simulink model "V0_2_5_2025_11_18_FullFMS"  (R2025b)
settings: Solver=VariableStepAuto  StartTime=0.0  StopTime=inf  RelTol=1e-3
libraries: opcualib x8
(part 1 of 3)
settings Model: SimulationMode=accelerator  Creator=guilh  LastModifiedBy=guilh

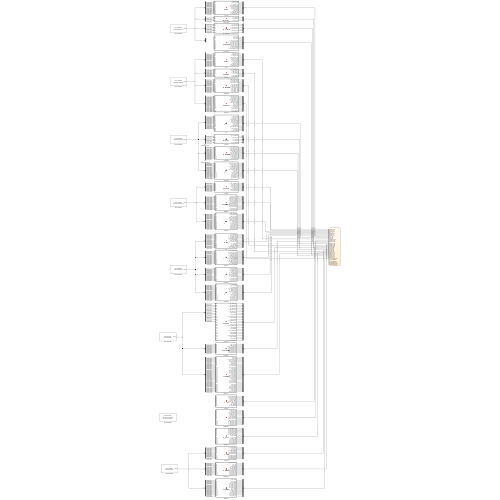
[thumbnail: Simulink's stored preview of the top-level diagram]
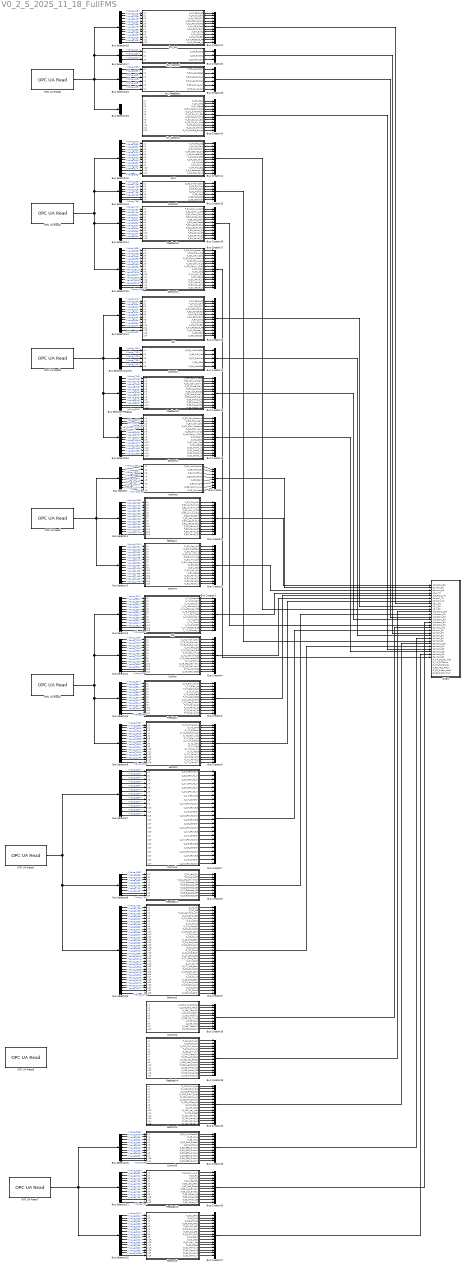
== system V0_2_5_2025_11_18_FullFMS ==
  ASI : MATLAB Function  TreatAsAtomicUnit=on
  Asi : MATLAB Function  TreatAsAtomicUnit=on
  Asi1 : MATLAB Function  TreatAsAtomicUnit=on
  Bus Creator : BusCreator  Inputs=8
  Bus Creator1 : BusCreator  Inputs=13
  Bus Creator10 : BusCreator  Inputs=14
  Bus Creator11 : BusCreator  Inputs=5
  Bus Creator{5,12,14,16,21,24,26} (7 alike) : BusCreator  Inputs=12
  Bus Creator{2,6,13,17,20} (5 alike) : BusCreator  Inputs=15
  Bus Creator15 : BusCreator  Inputs=7
  Bus Creator18 : BusCreator  Inputs=10
  Bus Creator19 : BusCreator  Inputs=14
  Bus Creator22 : BusCreator  Inputs=3
  Bus Creator23 : BusCreator  Inputs=6
  Bus Creator25 : BusCreator  Inputs=11
  Bus Creator27 : BusCreator  Inputs=16
  Bus Creator3 : BusCreator  Inputs=13
  Bus Creator4 : BusCreator  Inputs=13
  Bus Creator7 : BusCreator  Inputs=24
  Bus Creator8 : BusCreator  Inputs=9
  Bus Creator9 : BusCreator  Inputs=33
  Bus Selector : BusSelector  OutputSignals=Value_1062,Value_1072,Value_1082,Value_1094,Value_1104,Value_1114,Value_1124,Value_1134
  Bus Selector/Control : BusSelector  OutputSignals=Value_700,Value_710,Value_720,Value_730,Value_740
  Bus Selector/Feedback : BusSelector  OutputSignals=Value_756,Value_766,Value_776,Value_786,Value_796,Value_806,Value_816,Value_826,Value_836,Value_846,Value_856,Value_866
  Bus Selector1 : BusSelector  OutputSignals=Value_1150,Value_1160,Value_1170,Value_1180,Value_1190,Value_1200,Value_1210,Value_1220,Value_1230,Value_1240,Value_1250,Value_1260,Value_1270
  Bus Selector10 : BusSelector  OutputSignals=Value_885,Value_898,Value_913,Value_926,Value_939,Value_952,Value_965,Value_978,Value_991,Value_1004,Value_1017,Value_1030,Value_1043,Value_1056,Value_1069
  Bus Selector11 : BusSelector  OutputSignals=Value_574,Value_584,Value_594,Value_604,Value_614,Value_624,Value_634,Value_644,Value_654,Value_664,Value_674,Value_684
  Bus Selector12 : BusSelector  OutputSignals=Value_572,Value_582,Value_592,Value_602,Value_612,Value_622,Value_632,Value_642,Value_652,Value_662,Value_672,Value_682
  Bus Selector13 : BusSelector  OutputSignals=Value_698,Value_708,Value_718,Value_728,Value_738,Value_748,Value_758
  Bus Selector14 : BusSelector  OutputSignals=Value_774,Value_784,Value_794,Value_804,Value_814,Value_824,Value_834,Value_844,Value_854,Value_864,Value_874,Value_884
  Bus Selector15 : BusSelector  OutputSignals=Value_905,Value_918,Value_933,Value_946,Value_959,Value_972,Value_985,Value_998,Value_1011,Value_1024,Value_1037,Value_1050,Value_1063,Value_1076,Value_1089
  Bus Selector16 : BusSelector  OutputSignals=Value_215,Value_225,Value_235,Value_245,Value_255,Value_265,Value_275,Value_285,Value_295,Value_305,Value_315,Value_325
  Bus Selector17 : BusSelector  OutputSignals=Value_341,Value_354,Value_367
  Bus Selector18 : BusSelector  OutputSignals=Value_383,Value_393,Value_403,Value_413,Value_423,Value_433
  Bus Selector19 : BusSelector  OutputSignals=signal1,signal2
  Bus Selector2 : BusSelector  OutputSignals=Value_1291,Value_1304,Value_1319,Value_1332,Value_1345,Value_1358,Value_1371,Value_1384,Value_1397,Value_1410,Value_1423,Value_1436,Value_1449,Value_1462,Value_1475
  Bus Selector20 : BusSelector  OutputSignals=Value_566,Value_576,Value_586,Value_596,Value_606,Value_616,Value_626,Value_636,Value_646,Value_656,Value_666
  Bus Selector21 : BusSelector  OutputSignals=Value_682,Value_692,Value_702,Value_712,Value_722,Value_732,Value_742,Value_752,Value_762,Value_772,Value_782,Value_792
  Bus Selector22 : BusSelector  OutputSignals=Value_811,Value_824,Value_839,Value_852,Value_865,Value_878,Value_891,Value_904,Value_917,Value_930,Value_943,Value_956,Value_969,Value_982,Value_995,Value_1008
  Bus Selector3 : BusSelector  OutputSignals=Value_572,Value_582,Value_592,Value_602,Value_612,Value_622,Value_632,Value_642,Value_652,Value_662,Value_672,Value_682,Value_692
  Bus Selector4 : BusSelector  OutputSignals=Value_708,Value_718,Value_728,Value_738,Value_748,Value_758,Value_768,Value_778,Value_788,Value_798,Value_808,Value_818,Value_828
  Bus Selector5 : BusSelector  OutputSignals=Value_844,Value_854,Value_864,Value_874,Value_884,Value_894,Value_904,Value_914,Value_924,Value_934,Value_944,Value_954
  Bus Selector6 : BusSelector  OutputSignals=Value_975,Value_988,Value_1003,Value_1016,Value_1029,Value_1042,Value_1055,Value_1068,Value_1081,Value_1094,Value_1107,Value_1120,Value_1133,Value_1146,Value_1159
  Bus Selector7 : BusSelector  OutputSignals=Value_527,Value_537,Value_547,Value_557,Value_567,Value_577,Value_587,Value_597,Value_607,Value_617,Value_627,Value_637
  Bus Selector8 : BusSelector  OutputSignals=Value_653,Value_663,Value_673,Value_683,Value_693,Value_703,Value_713,Value_723,Value_733
  Bus Selector9 : BusSelector  OutputSignals=Value_752,Value_765,Value_780,Value_793,Value_806,Value_819,Value_832,Value_845,Value_858,Value_871,Value_884,Value_897,Value_910,Value_923,Value_936,Value_949,Value_962,Value_975,Value_988,Value_1001,Value_1014,Value_1027,Value_1040,Value_1053,Value_1066,Value_1079,Value_1092,Value_1105,Value_1118,Value_1131,Value_1144,Value_1157,Value_1170
  Chart : Stateflow chart  TreatAsAtomicUnit=on
      settings: PortSchema="{\"entries\":[{\"content\":{\"sides\":[{\"content\":{\"connectorIds\":[\"In2\",\"In1\",\"In3\",\"In4\",\"In6\",\"In5\",\"In7\",\"In8\",\"In9\",\"In10\",\"In11\",\"In12\",\"In13\",\"In14\",\"In15\",\"In16\",\"In17\",\"In18\",\"In19\",\"In20\",\"In21\",\"In22\",\"In23\",\"In24\",\"In25\",\"In26\",\"In27\",\"In28\",\"In29\",\"In30\",\"In31\",\"In32\",\"In33\",\"In34\"]},\"type\":\"ConnectorPlacement.EquallySpacedRectSide\",\"uuid\":\"e54bf7d4-7c7d-41d9-a8b8-f479ac319a99\"},{\"content\":{\"side\":\"RIGHT\"},\"type\":\"ConnectorPlacement.EquallySpacedRectSide\",\"uuid\":\"d3c20706-71bd-4e26-b40f-0ee7e71b06ee\"},{\"content\":{\"side\":\"TOP\"},\"type\":\"ConnectorPlacement.EquallySpacedRectSide\",\"uuid\":\"ecfb6920-e95b-4ed8-99f9-df5ce878328e\"}]},\"type\":\"ConnectorPlacement.EquallySpacedConnector\",\"uuid\":\"2e714192-4eea-4e1a-8945-7c827feed48f\"}],\"packageUris\":[\"http://schema.mathworks.com/mf0/Connector/R2020b\"],\"version\":\"1.0\"}"
  Control : MATLAB Function  TreatAsAtomicUnit=on
  Control1 : MATLAB Function  TreatAsAtomicUnit=on
  Control2 : MATLAB Function  TreatAsAtomicUnit=on
  Control3 : MATLAB Function  TreatAsAtomicUnit=on
  Control4 : MATLAB Function  TreatAsAtomicUnit=on
  Control5 : MATLAB Function  TreatAsAtomicUnit=on
  Feedback : MATLAB Function  TreatAsAtomicUnit=on
  Feedback1 : MATLAB Function  TreatAsAtomicUnit=on
  Feedback2 : MATLAB Function  TreatAsAtomicUnit=on
  Feedback3 : MATLAB Function  TreatAsAtomicUnit=on
  Feedback4 : MATLAB Function  TreatAsAtomicUnit=on
  Feedback5 : MATLAB Function  TreatAsAtomicUnit=on
  OPC UA Read : opcualib/OPC UA Read  SelectedServer=AAS OPC Distribution  ServerList=AAS OPC Distribution  NodeList={ '1', 'Value', '6', '1062', '1'; '2', 'Value', '6', '1072', '1'; '3', 'Value', '6', '1082', '1'; '4', 'Value', '6', '1094', '1'; '5', 'Value', '6', '1104', '1'; '6', 'Value', '6', '1114', '1'; '7', 'Value', '6', '1124', '1'; '8', 'Value', '6', '1134', '1'; '9', 'Value', '6', '1150', '1'; '10', 'Value', '6', '1160', '1'; '11', 'Value', '6', '1170', '1'; '12', 'Value', '6', '1180', '1'; '13', 'Value', '6', '1190', '1'; '14', 'Value', '6', '1200', '1'; '15', 'Value', '6', '1210', '1'; '16', 'Value', '6', '1220', '1'; '17', 'Value', '6', '1230', '1'; '18', 'Value', '6', '1240', '1'; '19', 'Value', '6', '1250', '1'; '20', 'Value', '6', '1260', '1'; '21', 'Value', '6', '1270', '1'; '22', 'Value', '6', '1291', '1'; '23', 'Value', '6', '1304', '1'; '24', 'Value', '6', '1319', '1'; '25', 'Value', '6', '1332', '1'; '26', 'Value', '6', '1345', '1'; '27', 'Value', '6', '1358', '1'; '28', 'Value', '6', '1371', '1'; '29', 'Value', '6', '1384', '1'; '30', 'Value', '6', '1397', '1'; '31', 'Value', '6', '1410', '1'; '32', 'Value', '6', '1423', '1'; '33', 'Value', '6', '1436', '1'; '34', 'Value', '6', '1449', '1'; '35', 'Value', '6', '1462', '1'; '36', 'Value', '6', '1475', '1' }  ShowQualityPort=off  ShowTimestampPort=off  ShowTimestampPortAs=Seconds since start  SampleTime=-1
  OPC UA Read1 : opcualib/OPC UA Read  SelectedServer=AAS OPC Testing  ServerList=AAS OPC Testing  NodeList={ '1', 'Value', '6', '572', '1'; '2', 'Value', '6', '582', '1'; '3', 'Value', '6', '592', '1'; '4', 'Value', '6', '602', '1'; '5', 'Value', '6', '612', '1'; '6', 'Value', '6', '622', '1'; '7', 'Value', '6', '632', '1'; '8', 'Value', '6', '642', '1'; '9', 'Value', '6', '652', '1'; '10', 'Value', '6', '662', '1'; '11', 'Value', '6', '672', '1'; '12', 'Value', '6', '682', '1'; '13', 'Value', '6', '692', '1'; '14', 'Value', '6', '708', '1'; '15', 'Value', '6', '718', '1'; '16', 'Value', '6', '728', '1'; '17', 'Value', '6', '738', '1'; '18', 'Value', '6', '748', '1'; '19', 'Value', '6', '758', '1'; '20', 'Value', '6', '768', '1'; '21', 'Value', '6', '778', '1'; '22', 'Value', '6', '788', '1'; '23', 'Value', '6', '798', '1'; '24', 'Value', '6', '808', '1'; '25', 'Value', '6', '818', '1'; '26', 'Value', '6', '828', '1'; '27', 'Value', '6', '844', '1'; '28', 'Value', '6', '854', '1'; '29', 'Value', '6', '864', '1'; '30', 'Value', '6', '874', '1'; '31', 'Value', '6', '884', '1'; '32', 'Value', '6', '894', '1'; '33', 'Value', '6', '904', '1'; '34', 'Value', '6', '914', '1'; '35', 'Value', '6', '924', '1'; '36', 'Value', '6', '934', '1'; '37', 'Value', '6', '944', '1'; '38', 'Value', '6', '954', '1'; '39', 'Value', '6', '975', '1'; '40', 'Value', '6', '988', '1'; '41', 'Value', '6', '1003', '1'; '42', 'Value', '6', '1016', '1'; '43', 'Value', '6', '1029', '1'; '44', 'Value', '6', '1042', '1'; '45', 'Value', '6', '1055', '1'; '46', 'Value', '6', '1068', '1'; '47', 'Value', '6', '1081', '1'; '48', 'Value', '6', '1094', '1'; '49', 'Value', '6', '1107', '1'; '50', 'Value', '6', '1120', '1'; '51', 'Value', '6', '1133', '1'; '52', 'Value', '6', '1146', '1'; '53', 'Value', '6', '1159', '1' }  ShowQualityPort=off  ShowTimestampPort=off  ShowTimestampPortAs=Seconds since start  SampleTime=-1
  OPC UA Read2 : opcualib/OPC UA Read  SelectedServer=AAS OPC Master  ServerList=AAS OPC Master  NodeList={ '1', 'Value', '6', '527', '1'; '2', 'Value', '6', '537', '1'; '3', 'Value', '6', '547', '1'; '4', 'Value', '6', '557', '1'; '5', 'Value', '6', '567', '1'; '6', 'Value', '6', '577', '1'; '7', 'Value', '6', '587', '1'; '8', 'Value', '6', '597', '1'; '9', 'Value', '6', '607', '1'; '10', 'Value', '6', '617', '1'; '11', 'Value', '6', '627', '1'; '12', 'Value', '6', '637', '1'; '13', 'Value', '6', '653', '1'; '14', 'Value', '6', '663', '1'; '15', 'Value', '6', '673', '1'; '16', 'Value', '6', '683', '1'; '17', 'Value', '6', '693', '1'; '18', 'Value', '6', '703', '1'; '19', 'Value', '6', '713', '1'; '20', 'Value', '6', '723', '1'; '21', 'Value', '6', '733', '1'; '22', 'Value', '6', '752', '1'; '23', 'Value', '6', '765', '1'; '24', 'Value', '6', '780', '1'; '25', 'Value', '6', '793', '1'; '26', 'Value', '6', '806', '1'; '27', 'Value', '6', '819', '1'; '28', 'Value', '6', '832', '1'; '29', 'Value', '6', '845', '1'; '30', 'Value', '6', '858', '1'; '31', 'Value', '6', '871', '1'; '32', 'Value', '6', '884', '1'; '33', 'Value', '6', '897', '1'; '34', 'Value', '6', '910', '1'; '35', 'Value', '6', '923', '1'; '36', 'Value', '6', '936', '1'; '37', 'Value', '6', '949', '1'; '38', 'Value', '6', '962', '1'; '39', 'Value', '6', '975', '1'; '40', 'Value', '6', '988', '1'; '41', 'Value', '6', '1001', '1'; '42', 'Value', '6', '1014', '1'; '43', 'Value', '6', '1027', '1'; '44', 'Value', '6', '1040', '1'; '45', 'Value', '6', '1053', '1'; '46', 'Value', '6', '1066', '1'; '47', 'Value', '6', '1079', '1'; '48', 'Value', '6', '1092', '1'; '49', 'Value', '6', '1105', '1'; '50', 'Value', '6', '1118', '1'; '51', 'Value', '6', '1131', '1'; '52', 'Value', '6', '1144', '1'; '53', 'Value', '6', '1157', '1'; '54', 'Value', '6', '1170', '1' }  ShowQualityPort=off  ShowTimestampPort=off  ShowTimestampPortAs=Seconds since start  SampleTime=-1
  OPC UA Read3 : opcualib/OPC UA Read  SelectedServer=AAS OPC Handling1  ServerList=AAS OPC Handling1  NodeList={ '1', 'Value', '6', '574', '1'; '2', 'Value', '6', '584', '1'; '3', 'Value', '6', '594', '1'; '4', 'Value', '6', '604', '1'; '5', 'Value', '6', '614', '1'; '6', 'Value', '6', '624', '1'; '7', 'Value', '6', '634', '1'; '8', 'Value', '6', '644', '1'; '9', 'Value', '6', '654', '1'; '10', 'Value', '6', '664', '1'; '11', 'Value', '6', '674', '1'; '12', 'Value', '6', '684', '1'; '13', 'Value', '6', '700', '1'; '14', 'Value', '6', '710', '1'; '15', 'Value', '6', '720', '1'; '16', 'Value', '6', '730', '1'; '17', 'Value', '6', '740', '1'; '18', 'Value', '6', '756', '1'; '19', 'Value', '6', '766', '1'; '20', 'Value', '6', '776', '1'; '21', 'Value', '6', '786', '1'; '22', 'Value', '6', '796', '1'; '23', 'Value', '6', '806', '1'; '24', 'Value', '6', '816', '1'; '25', 'Value', '6', '826', '1'; '26', 'Value', '6', '836', '1'; '27', 'Value', '6', '846', '1'; '28', 'Value', '6', '856', '1'; '29', 'Value', '6', '866', '1'; '30', 'Value', '6', '885', '1'; '31', 'Value', '6', '898', '1'; '32', 'Value', '6', '913', '1'; '33', 'Value', '6', '926', '1'; '34', 'Value', '6', '939', '1'; '35', 'Value', '6', '952', '1'; '36', 'Value', '6', '965', '1'; '37', 'Value', '6', '978', '1'; '38', 'Value', '6', '991', '1'; '39', 'Value', '6', '1004', '1'; '40', 'Value', '6', '1017', '1'; '41', 'Value', '6', '1030', '1'; '42', 'Value', '6', '1043', '1'; '43', 'Value', '6', '1056', '1'; '44', 'Value', '6', '1069', '1' }  ShowQualityPort=off  ShowTimestampPort=off  ShowTimestampPortAs=Seconds since start  SampleTime=-1
  OPC UA Read4 : opcualib/OPC UA Read  SelectedServer=AAS OPC Handling2  ServerList=AAS OPC Handling2  NodeList={ '1', 'Value', '6', '572', '1'; '2', 'Value', '6', '582', '1'; '3', 'Value', '6', '592', '1'; '4', 'Value', '6', '602', '1'; '5', 'Value', '6', '612', '1'; '6', 'Value', '6', '622', '1'; '7', 'Value', '6', '632', '1'; '8', 'Value', '6', '642', '1'; '9', 'Value', '6', '652', '1'; '10', 'Value', '6', '662', '1'; '11', 'Value', '6', '672', '1'; '12', 'Value', '6', '682', '1'; '13', 'Value', '6', '698', '1'; '14', 'Value', '6', '708', '1'; '15', 'Value', '6', '718', '1'; '16', 'Value', '6', '728', '1'; '17', 'Value', '6', '738', '1'; '18', 'Value', '6', '748', '1'; '19', 'Value', '6', '758', '1'; '20', 'Value', '6', '774', '1'; '21', 'Value', '6', '784', '1'; '22', 'Value', '6', '794', '1'; '23', 'Value', '6', '804', '1'; '24', 'Value', '6', '814', '1'; '25', 'Value', '6', '824', '1'; '26', 'Value', '6', '834', '1'; '27', 'Value', '6', '844', '1'; '28', 'Value', '6', '854', '1'; '29', 'Value', '6', '864', '1'; '30', 'Value', '6', '874', '1'; '31', 'Value', '6', '884', '1'; '32', 'Value', '6', '905', '1'; '33', 'Value', '6', '918', '1'; '34', 'Value', '6', '933', '1'; '35', 'Value', '6', '946', '1'; '36', 'Value', '6', '959', '1'; '37', 'Value', '6', '972', '1'; '38', 'Value', '6', '985', '1'; '39', 'Value', '6', '998', '1'; '40', 'Value', '6', '1011', '1'; '41', 'Value', '6', '1024', '1'; '42', 'Value', '6', '1037', '1'; '43', 'Value', '6', '1050', '1'; '44', 'Value', '6', '1063', '1'; '45', 'Value', '6', '1076', '1'; '46', 'Value', '6', '1089', '1' }  ShowQualityPort=off  ShowTimestampPort=off  ShowTimestampPortAs=Seconds since start  SampleTime=-1
  OPC UA Read5 : opcualib/OPC UA Read  SelectedServer=AAS OPC Processing  ServerList=AAS OPC Processing  NodeList={}  ShowQualityPort=on  ShowTimestampPort=on  ShowTimestampPortAs=Seconds since start  SampleTime=-1
  OPC UA Read6 : opcualib/OPC UA Read  SelectedServer=Node-RED OPCUA  ServerList=Node-RED OPCUA  NodeList={ '1', 'Value', '6', '215', '1'; '2', 'Value', '6', '225', '1'; '3', 'Value', '6', '235', '1'; '4', 'Value', '6', '245', '1'; '5', 'Value', '6', '255', '1'; '6', 'Value', '6', '265', '1'; '7', 'Value', '6', '275', '1'; '8', 'Value', '6', '285', '1'; '9', 'Value', '6', '295', '1'; '10', 'Value', '6', '305', '1'; '11', 'Value', '6', '315', '1'; '12', 'Value', '6', '325', '1'; '13', 'Value', '6', '341', '1'; '14', 'Value', '6', '354', '1'; '15', 'Value', '6', '367', '1'; '16', 'Value', '6', '383', '1'; '17', 'Value', '6', '393', '1'; '18', 'Value', '6', '403', '1'; '19', 'Value', '6', '413', '1'; '20', 'Value', '6', '423', '1'; '21', 'Value', '6', '433', '1' }  ShowQualityPort=off  ShowTimestampPort=off  ShowTimestampPortAs=Seconds since start  SampleTime=-1
  OPC UA Read7 : opcualib/OPC UA Read  SelectedServer=AAS OPC Sorting  ServerList=AAS OPC Sorting  NodeList={ '1', 'Value', '6', '566', '1'; '2', 'Value', '6', '576', '1'; '3', 'Value', '6', '586', '1'; '4', 'Value', '6', '596', '1'; '5', 'Value', '6', '606', '1'; '6', 'Value', '6', '616', '1'; '7', 'Value', '6', '626', '1'; '8', 'Value', '6', '636', '1'; '9', 'Value', '6', '646', '1'; '10', 'Value', '6', '656', '1'; '11', 'Value', '6', '666', '1'; '12', 'Value', '6', '682', '1'; '13', 'Value', '6', '692', '1'; '14', 'Value', '6', '702', '1'; '15', 'Value', '6', '712', '1'; '16', 'Value', '6', '722', '1'; '17', 'Value', '6', '732', '1'; '18', 'Value', '6', '742', '1'; '19', 'Value', '6', '752', '1'; '20', 'Value', '6', '762', '1'; '21', 'Value', '6', '772', '1'; '22', 'Value', '6', '782', '1'; '23', 'Value', '6', '792', '1'; '24', 'Value', '6', '811', '1'; '25', 'Value', '6', '824', '1'; '26', 'Value', '6', '839', '1'; '27', 'Value', '6', '852', '1'; '28', 'Value', '6', '865', '1'; '29', 'Value', '6', '878', '1'; '30', 'Value', '6', '891', '1'; '31', 'Value', '6', '904', '1'; '32', 'Value', '6', '917', '1'; '33', 'Value', '6', '930', '1'; '34', 'Value', '6', '943', '1'; '35', 'Value', '6', '956', '1'; '36', 'Value', '6', '969', '1'; '37', 'Value', '6', '982', '1'; '38', 'Value', '6', '995', '1'; '39', 'Value', '6', '1008', '1' }  ShowQualityPort=off  ShowTimestampPort=off  ShowTimestampPortAs=Seconds since start  SampleTime=-1
  Sensors : MATLAB Function  TreatAsAtomicUnit=on
  Sensors1 : MATLAB Function  TreatAsAtomicUnit=on
  Sensors2 : MATLAB Function  TreatAsAtomicUnit=on
  Sensors3 : MATLAB Function  TreatAsAtomicUnit=on
  Sensors4 : MATLAB Function  TreatAsAtomicUnit=on
  Sensors5 : MATLAB Function  TreatAsAtomicUnit=on
  controls : MATLAB Function  TreatAsAtomicUnit=on
  fcn_Asi : MATLAB Function  TreatAsAtomicUnit=on
  fcn_Control : MATLAB Function  TreatAsAtomicUnit=on
  fcn_Feedback : MATLAB Function  TreatAsAtomicUnit=on
  fcn_Sensors : MATLAB Function  TreatAsAtomicUnit=on
  feedback : MATLAB Function  TreatAsAtomicUnit=on
  sensors : MATLAB Function  TreatAsAtomicUnit=on
  wires:
  OPC UA Read/1 -> Bus Selector2/1, Bus Selector/1, Bus Selector1/1
  Bus Selector/1 -> controls/1(u1)  "<Value_1062>"
  Bus Selector/2 -> controls/2(u2)  "<Value_1072>"
  Bus Selector/3 -> controls/3(u3)  "<Value_1082>"
  Bus Selector/4 -> controls/4(u4)  "<Value_1094>"
  Bus Selector/5 -> controls/5(u5)  "<Value_1104>"
  Bus Selector/6 -> controls/6(u6)  "<Value_1114>"
  Bus Selector/7 -> controls/7(u7)  "<Value_1124>"
  Bus Selector/8 -> controls/8(u8)  "<Value_1134>"
  Bus Selector1/11 -> feedback/11(u11)  "<Value_1250>"
  Bus Selector1/12 -> feedback/12(u12)  "<Value_1260>"
  Bus Selector1/13 -> feedback/13(u13)  "<Value_1270>"
  Bus Selector1/1 -> feedback/1(u1)  "<Value_1150>"
  Bus Selector1/2 -> feedback/2(u2)  "<Value_1160>"
  Bus Selector1/3 -> feedback/3(u3)  "<Value_1170>"
  Bus Selector1/4 -> feedback/4(u4)  "<Value_1180>"
  Bus Selector1/5 -> feedback/5(u5)  "<Value_1190>"
  Bus Selector1/6 -> feedback/6(u6)  "<Value_1200>"
  Bus Selector1/7 -> feedback/7(u7)  "<Value_1210>"
  Bus Selector1/8 -> feedback/8(u8)  "<Value_1220>"
  Bus Selector1/9 -> feedback/9(u9)  "<Value_1230>"
  Bus Selector1/10 -> feedback/10(u10)  "<Value_1240>"
  Bus Selector2/1 -> sensors/1(u1)  "<Value_1291>"
  Bus Selector2/2 -> sensors/2(u2)  "<Value_1304>"
  Bus Selector2/3 -> sensors/3(u3)  "<Value_1319>"
  Bus Selector2/4 -> sensors/4(u4)  "<Value_1332>"
  Bus Selector2/5 -> sensors/5(u5)  "<Value_1345>"
  Bus Selector2/6 -> sensors/6(u6)  "<Value_1358>"
  Bus Selector2/7 -> sensors/7(u7)  "<Value_1371>"
  Bus Selector2/8 -> sensors/8(u8)  "<Value_1384>"
  Bus Selector2/9 -> sensors/9(u9)  "<Value_1397>"
  Bus Selector2/10 -> sensors/10(u10)  "<Value_1410>"
  Bus Selector2/11 -> sensors/11(u11)  "<Value_1423>"
  Bus Selector2/12 -> sensors/12(u12)  "<Value_1436>"
  Bus Selector2/13 -> sensors/13(u13)  "<Value_1449>"
  Bus Selector2/14 -> sensors/14(u14)  "<Value_1462>"
  Bus Selector2/15 -> sensors/15(u15)  "<Value_1475>"
  OPC UA Read1/1 -> Bus Selector6/1, Bus Selector5/1, Bus Selector3/1, Bus Selector4/1
  Bus Selector3/1 -> ASI/1(u1)  "<Value_572>"
  Bus Selector3/2 -> ASI/2(u2)  "<Value_582>"
  Bus Selector3/3 -> ASI/3(u3)  "<Value_592>"
  Bus Selector3/4 -> ASI/4(u4)  "<Value_602>"
  Bus Selector3/5 -> ASI/5(u5)  "<Value_612>"
  Bus Selector3/6 -> ASI/6(u6)  "<Value_622>"
  Bus Selector3/7 -> ASI/7(u7)  "<Value_632>"
  Bus Selector3/8 -> ASI/8(u8)  "<Value_642>"
  Bus Selector3/9 -> ASI/9(u9)  "<Value_652>"
  Bus Selector3/10 -> ASI/10(u10)  "<Value_662>"
  Bus Selector3/11 -> ASI/11(u11)  "<Value_672>"
  Bus Selector3/12 -> ASI/12(u12)  "<Value_682>"
  Bus Selector3/13 -> ASI/13(u13)  "<Value_692>"
  Bus Selector4/1 -> Control/1(u1)  "<Value_708>"
  Bus Selector4/2 -> Control/2(u2)  "<Value_718>"
  Bus Selector4/3 -> Control/3(u3)  "<Value_728>"
  Bus Selector4/4 -> Control/4(u4)  "<Value_738>"
  Bus Selector4/5 -> Control/5(u5)  "<Value_748>"
  Bus Selector4/6 -> Control/6(u6)  "<Value_758>"
  Bus Selector4/7 -> Control/7(u7)  "<Value_768>"
  Bus Selector4/8 -> Control/8(u8)  "<Value_778>"
  Bus Selector4/9 -> Control/9(u9)  "<Value_788>"
  Bus Selector4/10 -> Control/10(u10)  "<Value_798>"
  Bus Selector4/11 -> Control/11(u11)  "<Value_808>"
  Bus Selector4/12 -> Control/12(u12)  "<Value_818>"
  Bus Selector4/13 -> Control/13(u13)  "<Value_828>"
  Bus Selector5/1 -> Feedback/1(u1)  "<Value_844>"
  Bus Selector5/2 -> Feedback/2(u2)  "<Value_854>"
  Bus Selector5/3 -> Feedback/3(u3)  "<Value_864>"
  Bus Selector5/4 -> Feedback/4(u4)  "<Value_874>"
  Bus Selector5/5 -> Feedback/5(u5)  "<Value_884>"
  Bus Selector5/6 -> Feedback/6(u6)  "<Value_894>"
  Bus Selector5/7 -> Feedback/7(u7)  "<Value_904>"
  Bus Selector5/8 -> Feedback/8(u8)  "<Value_914>"
  Bus Selector5/9 -> Feedback/9(u9)  "<Value_924>"
  Bus Selector5/10 -> Feedback/10(u10)  "<Value_934>"
  Bus Selector5/11 -> Feedback/11(u11)  "<Value_944>"
  Bus Selector5/12 -> Feedback/12(u12)  "<Value_954>"
  Bus Selector6/1 -> Sensors/1(u1)  "<Value_975>"
  Bus Selector6/2 -> Sensors/2(u2)  "<Value_988>"
  Bus Selector6/3 -> Sensors/3(u3)  "<Value_1003>"
  Bus Selector6/4 -> Sensors/4(u4)  "<Value_1016>"
  Bus Selector6/5 -> Sensors/5(u5)  "<Value_1029>"
  Bus Selector6/6 -> Sensors/6(u6)  "<Value_1042>"
  Bus Selector6/7 -> Sensors/7(u7)  "<Value_1055>"
  Bus Selector6/8 -> Sensors/8(u8)  "<Value_1068>"
  Bus Selector6/9 -> Sensors/9(u9)  "<Value_1081>"
  Bus Selector6/10 -> Sensors/10(u10)  "<Value_1094>"
  Bus Selector6/11 -> Sensors/11(u11)  "<Value_1107>"
  Bus Selector6/12 -> Sensors/12(u12)  "<Value_1120>"
  Bus Selector6/13 -> Sensors/13(u13)  "<Value_1133>"
  Bus Selector6/14 -> Sensors/14(u14)  "<Value_1146>"
  Bus Selector6/15 -> Sensors/15(u15)  "<Value_1159>"
  controls/1(C_85_Initialization) -> Bus Creator/1
  controls/2(C_85_Part_Del) -> Bus Creator/2
  controls/3(C_82_Profibus) -> Bus Creator/3
  controls/4(C_83_RQ_Parts) -> Bus Creator/4
  controls/5(C_85_Start) -> Bus Creator/5
  controls/6(C_85_Single) -> Bus Creator/6
  controls/7(C_85_Continuous) -> Bus Creator/7
  controls/8(C_85_Counted) -> Bus Creator/8
  feedback/1(F_82_Pist_Adv) -> Bus Creator1/1
  feedback/2(F_82_Suction_On) -> Bus Creator1/2
  feedback/3(F_82_Suction_Off) -> Bus Creator1/3
  feedback/4(F_82_Arm_2_Del) -> Bus Creator1/4
  feedback/5(F_82_Arm_2_Mag) -> Bus Creator1/5
  feedback/6(F_83_Led_Start) -> Bus Creator1/6
  feedback/7(F_83_Led_Reset) -> Bus Creator1/7
  feedback/8(F_83_Led_Extra1) -> Bus Creator1/8
  feedback/9(F_83_Led_Extra2) -> Bus Creator1/9
  feedback/10(F_83_Panel_O4) -> Bus Creator1/10
  feedback/11(F_83_Panel_O5) -> Bus Creator1/11
  feedback/12(F_83_Panel_O6) -> Bus Creator1/12
  feedback/13(F_83_Panel_O7) -> Bus Creator1/13
  sensors/1(O_80_Mag_Full) -> Bus Creator2/1
  sensors/2(O_80_Pist_Back) -> Bus Creator2/2
  sensors/3(O_80_Pist_Fwd) -> Bus Creator2/3
  sensors/4(O_80_Part_Stuck) -> Bus Creator2/4
  sensors/5(O_80_Arm_Mag) -> Bus Creator2/5
  sensors/6(O_80_Arm_Del) -> Bus Creator2/6
  sensors/7(O_80_Mag_Empty) -> Bus Creator2/7
  sensors/8(O_81_Start) -> Bus Creator2/8
  sensors/9(O_81_Stop) -> Bus Creator2/9
  sensors/10(O_81_Key_Pos) -> Bus Creator2/10
  sensors/11(O_81_Reset) -> Bus Creator2/11
  sensors/12(O_81_Panel_I4) -> Bus Creator2/12
  sensors/13(O_81_Panel_I5) -> Bus Creator2/13
  sensors/14(O_81_Panel_I6) -> Bus Creator2/14
  sensors/15(O_81_Panel_I7) -> Bus Creator2/15
  ASI/1(A_74_Request) -> Bus Creator3/1
  ASI/2(A_74_No_Cart) -> Bus Creator3/2
  ASI/3(A_74_Cart_Full) -> Bus Creator3/3
  ASI/4(A_74_CRoute_Out) -> Bus Creator3/4
  ASI/5(A_74_CRoute_In80) -> Bus Creator3/5
  ASI/6(A_73_TestCartID) -> Bus Creator3/6
  ASI/7(A_74_Cart_Stat) -> Bus Creator3/7
  ASI/8(A_74_Cart_Next) -> Bus Creator3/8
  ASI/9(A_74_Optic) -> Bus Creator3/9
  ASI/10(A_74_Count) -> Bus Creator3/10
  ASI/11(A_74_Pist_Bck) -> Bus Creator3/11
  ASI/12(A_74_Release_FB) -> Bus Creator3/12
  ASI/13(A_74_CRoute_In) -> Bus Creator3/13
  Control/1(C_75_Initialization) -> Bus Creator4/1
  Control/2(C_75_ID_Delivery1) -> Bus Creator4/2
  Control/3(C_75_ID_Delivery2) -> Bus Creator4/3
  Control/4(C_75_Part_Del) -> Bus Creator4/4
  Control/5(C_75_RQ_Part_Del) -> Bus Creator4/5
  Control/6(C_75_RQ_Wrong) -> Bus Creator4/6
  Control/7(C_75_Identified80) -> Bus Creator4/7
  Control/8(C_75_Requested80) -> Bus Creator4/8
  Control/9(C_72_Profibus) -> Bus Creator4/9
  Control/10(C_75_RQ_Delivery1) -> Bus Creator4/10
  Control/11(C_75_RQ_Delivery2) -> Bus Creator4/11
  Control/12(C_75_Identified) -> Bus Creator4/12
  Control/13(C_75_Requested) -> Bus Creator4/13
  Feedback/1(F_72_Elev_Down) -> Bus Creator5/1
  Feedback/2(F_72_Elev_Up) -> Bus Creator5/2
  Feedback/3(F_72_Eject_Part) -> Bus Creator5/3
  Feedback/4(F_72_Air_On) -> Bus Creator5/4
  Feedback/5(F_73_Led_Start) -> Bus Creator5/5
  Feedback/6(F_73_Led_Reset) -> Bus Creator5/6
  Feedback/7(F_73_Led_Extra1) -> Bus Creator5/7
  Feedback/8(F_73_Led_Extra2) -> Bus Creator5/8
  Feedback/9(F_73_Panel_O4) -> Bus Creator5/9
  Feedback/10(F_73_Panel_O5) -> Bus Creator5/10
  Feedback/11(F_73_Panel_O6) -> Bus Creator5/11
  Feedback/12(F_73_Panel_O7) -> Bus Creator5/12
  Sensors/1(O_70_SInductive) -> Bus Creator6/1
  Sensors/2(O_70_SPart) -> Bus Creator6/2
  Sensors/3(O_70_SStation) -> Bus Creator6/3
  Sensors/4(O_70_SPart_Height) -> Bus Creator6/4
  Sensors/5(O_70_Elev_High) -> Bus Creator6/5
  Sensors/6(O_70_Elev_Low) -> Bus Creator6/6
  Sensors/7(O_70_Pist_Back) -> Bus Creator6/7
  Sensors/8(O_71_Start) -> Bus Creator6/8
  Sensors/9(O_71_Stop) -> Bus Creator6/9
  Sensors/10(O_71_Key_Pos) -> Bus Creator6/10
  Sensors/11(O_71_Reset) -> Bus Creator6/11
  Sensors/12(O_71_Panel_I4) -> Bus Creator6/12
  Sensors/13(O_71_Panel_I5) -> Bus Creator6/13
  Sensors/14(O_71_Panel_I6) -> Bus Creator6/14
  Sensors/15(O_71_Panel_I7) -> Bus Creator6/15
  Bus Creator/1 -> Chart/1(Control_80)
  Bus Creator1/1 -> Chart/2(Actuators_80)
  Bus Creator2/1 -> Chart/3(Sensors_80)
  Bus Creator6/1 -> Chart/7(Sensors_70)
  Bus Creator5/1 -> Chart/6(Actuators_70)
  Bus Creator4/1 -> Chart/5(Control_70)
  Bus Creator3/1 -> Chart/4(AS_i_70)
  OPC UA Read2/1 -> Bus Selector9/1, Bus Selector8/1, Bus Selector7/1
  Bus Selector7/1 -> Control1/1(u1)  "<Value_527>"
  Bus Selector7/2 -> Control1/2(u2)  "<Value_537>"
  Bus Selector7/3 -> Control1/3(u3)  "<Value_547>"
  Bus Selector7/4 -> Control1/4(u4)  "<Value_557>"
  Bus Selector7/5 -> Control1/5(u5)  "<Value_567>"
  Bus Selector7/6 -> Control1/6(u6)  "<Value_577>"
  Bus Selector7/7 -> Control1/7(u7)  "<Value_587>"
  Bus Selector7/8 -> Control1/8(u8)  "<Value_597>"
  Bus Selector7/9 -> Control1/9(u9)  "<Value_607>"
  Bus Selector7/10 -> Control1/10(u10)  "<Value_617>"
  Bus Selector7/11 -> Control1/11(u11)  "<Value_627>"
  Bus Selector7/12 -> Control1/12(u12)  "<Value_637>"
  Bus Selector8/1 -> Feedback1/1(u1)  "<Value_653>"
  Bus Selector8/2 -> Feedback1/2(u2)  "<Value_663>"
  Bus Selector8/3 -> Feedback1/3(u3)  "<Value_673>"
  Bus Selector8/4 -> Feedback1/4(u4)  "<Value_683>"
  Bus Selector8/5 -> Feedback1/5(u5)  "<Value_693>"
  Bus Selector8/6 -> Feedback1/6(u6)  "<Value_703>"
  Bus Selector8/7 -> Feedback1/7(u7)  "<Value_713>"
  Bus Selector8/8 -> Feedback1/8(u8)  "<Value_723>"
  Bus Selector8/9 -> Feedback1/9(u9)  "<Value_733>"
  Bus Selector9/1 -> Sensors1/1(u1)  "<Value_752>"
  Bus Selector9/3 -> Sensors1/3(u3)  "<Value_780>"
  Bus Selector9/2 -> Sensors1/2(u2)  "<Value_765>"
  Bus Selector9/4 -> Sensors1/4(u4)  "<Value_793>"
  Bus Selector9/5 -> Sensors1/5(u5)  "<Value_806>"
  Bus Selector9/6 -> Sensors1/6(u6)  "<Value_819>"
  Bus Selector9/7 -> Sensors1/7(u7)  "<Value_832>"
  Bus Selector9/8 -> Sensors1/8(u8)  "<Value_845>"
  Bus Selector9/9 -> Sensors1/9(u9)  "<Value_858>"
  Bus Selector9/10 -> Sensors1/10(u10)  "<Value_871>"
  Bus Selector9/11 -> Sensors1/11(u11)  "<Value_884>"
  Bus Selector9/12 -> Sensors1/12(u12)  "<Value_897>"
  Bus Selector9/13 -> Sensors1/13(u13)  "<Value_910>"
  Bus Selector9/14 -> Sensors1/14(u14)  "<Value_923>"
  Bus Selector9/15 -> Sensors1/15(u15)  "<Value_936>"
  Bus Selector9/16 -> Sensors1/16(u16)  "<Value_949>"
  Bus Selector9/17 -> Sensors1/17(u17)  "<Value_962>"
  Bus Selector9/18 -> Sensors1/18(u18)  "<Value_975>"
  Bus Selector9/19 -> Sensors1/19(u19)  "<Value_988>"
  Bus Selector9/20 -> Sensors1/20(u20)  "<Value_1001>"
  Bus Selector9/21 -> Sensors1/21(u21)  "<Value_1014>"
  Bus Selector9/22 -> Sensors1/22(u22)  "<Value_1027>"
  Bus Selector9/23 -> Sensors1/23(u23)  "<Value_1040>"
  Bus Selector9/24 -> Sensors1/24(u24)  "<Value_1053>"
  Bus Selector9/25 -> Sensors1/25(u25)  "<Value_1066>"
  Bus Selector9/26 -> Sensors1/26(u26)  "<Value_1079>"
  Bus Selector9/27 -> Sensors1/27(u27)  "<Value_1092>"
  Bus Selector9/28 -> Sensors1/28(u28)  "<Value_1105>"
  Bus Selector9/29 -> Sensors1/29(u29)  "<Value_1118>"
  Bus Selector9/30 -> Sensors1/30(u30)  "<Value_1131>"
  Bus Selector9/31 -> Sensors1/31(u31)  "<Value_1144>"
  Bus Selector9/32 -> Sensors1/32(u32)  "<Value_1157>"
  Bus Selector9/33 -> Sensors1/33(u33)  "<Value_1170>"
  Control1/1(C_24_CRoute_In) -> Bus Creator7/1
  Control1/2(C_25_CRoute_In) -> Bus Creator7/2
  Control1/3(C_26_CRoute_In) -> Bus Creator7/3
  Control1/4(C_27_CRoute_In) -> Bus Creator7/4
  Control1/5(C_28_CRoute_In) -> Bus Creator7/5
  Control1/6(C_29_CRoute_In) -> Bus Creator7/6
  Control1/7(C_24_Request) -> Bus Creator7/7
  Control1/8(C_24_CartDel) -> Bus Creator7/8
  Control1/9(C_24_CRoute_Out) -> Bus Creator7/9
  Control1/10(C_25_Request) -> Bus Creator7/10
  Control1/11(C_25_CartDel) -> Bus Creator7/11
  Control1/12(C_25_CRoute_Out) -> Bus Creator7/12
  Control1/13(C_26_Request) -> Bus Creator7/13
  Control1/14(C_26_CartDel) -> Bus Creator7/14
  Control1/15(C_26_CRoute_Out) -> Bus Creator7/15
  Control1/16(C_27_Request) -> Bus Creator7/16
  Control1/17(C_27_CartDel) -> Bus Creator7/17
  Control1/18(C_27_CRoute_Out) -> Bus Creator7/18
  Control1/19(C_28_Request) -> Bus Creator7/19
  Control1/20(C_28_CartDel) -> Bus Creator7/20
  Control1/21(C_28_CRoute_Out) -> Bus Creator7/21
  Control1/22(C_29_Request) -> Bus Creator7/22
  Control1/23(C_29_CartDel) -> Bus Creator7/23
  Control1/24(C_29_CRoute_Out) -> Bus Creator7/24
  Feedback1/1(F_22_Led_On) -> Bus Creator8/1
  Feedback1/2(F_22_Led_Off) -> Bus Creator8/2
  Feedback1/3(F_22_Led_Conveyor) -> Bus Creator8/3
  Feedback1/4(F_24_Release_FB) -> Bus Creator8/4
  Feedback1/5(F_25_Release_FB) -> Bus Creator8/5
  Feedback1/6(F_26_Release_FB) -> Bus Creator8/6
  Feedback1/7(F_27_Release_FB) -> Bus Creator8/7
  Feedback1/8(F_28_Release_FB) -> Bus Creator8/8
  Feedback1/9(F_29_Release_FB) -> Bus Creator8/9
  Sensors1/1(O_20_On) -> Bus Creator9/1
  Sensors1/2(O_20_Off) -> Bus Creator9/2
  Sensors1/3(O_20_Controler_On) -> Bus Creator9/3
  Sensors1/4(O_24_Cart_Stat) -> Bus Creator9/4
  Sensors1/5(O_24_Cart_Next) -> Bus Creator9/5
  Sensors1/6(O_24_Optic) -> Bus Creator9/6
  Sensors1/7(O_24_Count) -> Bus Creator9/7
  Sensors1/8(O_24_Pist_Bck) -> Bus Creator9/8
  Sensors1/9(O_25_Cart_Stat) -> Bus Creator9/9
  Sensors1/10(O_25_Cart_Next) -> Bus Creator9/10
  Sensors1/11(O_25_Optic) -> Bus Creator9/11
  Sensors1/12(O_25_Count) -> Bus Creator9/12
  Sensors1/13(O_25_Pist_Back) -> Bus Creator9/13
  Sensors1/14(O_26_Cart_Stat) -> Bus Creator9/14
  Sensors1/15(O_26_Cart_Next) -> Bus Creator9/15
  Sensors1/16(O_26_Optic) -> Bus Creator9/16
  Sensors1/17(O_26_Count) -> Bus Creator9/17
  Sensors1/18(O_26_Pist_Back) -> Bus Creator9/18
  Sensors1/19(O_27_Cart_Stat) -> Bus Creator9/19
  Sensors1/20(O_27_Cart_Next) -> Bus Creator9/20
  Sensors1/21(O_27_Optic) -> Bus Creator9/21
  Sensors1/22(O_27_Count) -> Bus Creator9/22
  Sensors1/23(O_27_Pist_Back) -> Bus Creator9/23
  Sensors1/24(O_28_Cart_Stat) -> Bus Creator9/24
  Sensors1/25(O_28_Cart_Next) -> Bus Creator9/25
  Sensors1/26(O_28_Optic) -> Bus Creator9/26
  Sensors1/27(O_28_Count) -> Bus Creator9/27
  Sensors1/28(O_28_Pist_Back) -> Bus Creator9/28
  Sensors1/29(O_29_Cart_Stat) -> Bus Creator9/29
  Sensors1/30(O_29_Cart_Next) -> Bus Creator9/30
  Sensors1/31(O_29_Optic) -> Bus Creator9/31
  Sensors1/32(O_29_Count) -> Bus Creator9/32
  Sensors1/33(O_29_Pist_Back) -> Bus Creator9/33
  Bus Creator7/1 -> Chart/18(Control_20)
  Bus Creator8/1 -> Chart/12(Actuators_20)
  Bus Creator9/1 -> Chart/24(Sensors_20)
  Bus Selector10/7 -> Sensors2/7(u7)  "<Value_965>"
  Bus Selector10/1 -> Sensors2/1(u1)  "<Value_885>"
  Bus Selector10/13 -> Sensors2/13(u13)  "<Value_1043>"
  Bus Selector10/2 -> Sensors2/2(u2)  "<Value_898>"
  Bus Selector10/4 -> Sensors2/4(u4)  "<Value_926>"
  Bus Selector10/8 -> Sensors2/8(u8)  "<Value_978>"
  Bus Selector10/15 -> Sensors2/15(u15)  "<Value_1069>"
  Bus Selector10/9 -> Sensors2/9(u9)  "<Value_991>"
  Bus Selector10/10 -> Sensors2/10(u10)  "<Value_1004>"
  Bus Selector10/11 -> Sensors2/11(u11)  "<Value_1017>"
  Bus Selector10/6 -> Sensors2/6(u6)  "<Value_952>"
  Bus Selector10/12 -> Sensors2/12(u12)  "<Value_1030>"
  Bus Selector10/14 -> Sensors2/14(u14)  "<Value_1056>"
  Bus Selector10/5 -> Sensors2/5(u5)  "<Value_939>"
  Bus Selector10/3 -> Sensors2/3(u3)  "<Value_913>"
  OPC UA Read3/1 -> Bus Selector10/1, Bus Selector/Feedback/1, Bus Selector/Control/1, Bus Selector11/1
  Bus Selector11/1 -> Asi/1(u1)  "<Value_574>"
  Bus Selector11/2 -> Asi/2(u2)  "<Value_584>"
  Bus Selector11/3 -> Asi/3(u3)  "<Value_594>"
  Bus Selector11/4 -> Asi/4(u4)  "<Value_604>"
  Bus Selector11/5 -> Asi/5(u5)  "<Value_614>"
  Bus Selector11/6 -> Asi/6(u6)  "<Value_624>"
  Bus Selector11/7 -> Asi/7(u7)  "<Value_634>"
  Bus Selector11/8 -> Asi/8(u8)  "<Value_644>"
  Bus Selector11/9 -> Asi/9(u9)  "<Value_654>"
  Bus Selector11/10 -> Asi/10(u10)  "<Value_664>"
  Bus Selector11/11 -> Asi/11(u11)  "<Value_674>"
  Bus Selector11/12 -> Asi/12(u12)  "<Value_684>"
  Bus Selector/Control/1 -> Control2/1(u1)  "<Value_700>"
  Bus Selector/Control/2 -> Control2/2(u2)  "<Value_710>"
  Bus Selector/Control/3 -> Control2/3(u3)  "<Value_720>"
  Bus Selector/Control/4 -> Control2/4(u4)  "<Value_730>"
  Bus Selector/Control/5 -> Control2/5(u5)  "<Value_740>"
  Bus Selector/Feedback/1 -> Feedback2/1(u1)  "<Value_756>"
  Bus Selector/Feedback/2 -> Feedback2/2(u2)  "<Value_766>"
  Bus Selector/Feedback/3 -> Feedback2/3(u3)  "<Value_776>"
  Bus Selector/Feedback/4 -> Feedback2/4(u4)  "<Value_786>"
  Bus Selector/Feedback/5 -> Feedback2/5(u5)  "<Value_796>"
  Bus Selector/Feedback/6 -> Feedback2/6(u6)  "<Value_806>"
  Bus Selector/Feedback/7 -> Feedback2/7(u7)  "<Value_816>"
  Bus Selector/Feedback/8 -> Feedback2/8(u8)  "<Value_826>"
  Bus Selector/Feedback/9 -> Feedback2/9(u9)  "<Value_836>"
  Bus Selector/Feedback/10 -> Feedback2/10(u10)  "<Value_846>"
  Bus Selector/Feedback/11 -> Feedback2/11(u11)  "<Value_856>"
  Bus Selector/Feedback/12 -> Feedback2/12(u12)  "<Value_866>"
  Sensors2/1(O_50_Part_Reserve) -> Bus Creator13/1
  Sensors2/2(O_50_Claw_Cart) -> Bus Creator13/2
  Sensors2/3(O_50_Claw_Del) -> Bus Creator13/3
  Sensors2/4(O_50_Claw_Reserve) -> Bus Creator13/4
  Sensors2/5(O_50_Claw_Low) -> Bus Creator13/5
  Sensors2/6(O_50_Claw_High) -> Bus Creator13/6
  Sensors2/7(O_50_Part_in_Claw) -> Bus Creator13/7
  Sensors2/8(O_51_Start) -> Bus Creator13/8
  Sensors2/9(O_51_Stop) -> Bus Creator13/9
  Sensors2/10(O_51_Key_Pos) -> Bus Creator13/10
  Sensors2/11(O_51_Reset) -> Bus Creator13/11
  Sensors2/12(O_51_Panel_I4) -> Bus Creator13/12
  Sensors2/13(O_51_Panel_I5) -> Bus Creator13/13
  Sensors2/14(O_51_Panel_I6) -> Bus Creator13/14
  Sensors2/15(O_51_Panel_I7) -> Bus Creator13/15
  Feedback2/1(F_52_Claw_2_Del) -> Bus Creator12/1
  Feedback2/2(F_52_Claw_2_Cart) -> Bus Creator12/2
  Feedback2/3(F_52_Claw_Down) -> Bus Creator12/3
  Feedback2/4(F_52_Close_Claw) -> Bus Creator12/4
  Feedback2/5(F_53_Led_Start) -> Bus Creator12/5
  Feedback2/6(F_53_Led_Reset) -> Bus Creator12/6
  Feedback2/7(F_53_Led_Extra1) -> Bus Creator12/7
  Feedback2/8(F_53_Led_Extra2) -> Bus Creator12/8
  Feedback2/9(F_53_Panel_O4) -> Bus Creator12/9
  Feedback2/10(F_53_Panel_O5) -> Bus Creator12/10
  Feedback2/11(F_53_Panel_O6) -> Bus Creator12/11
  Feedback2/12(F_53_Panel_O7) -> Bus Creator12/12
  Control2/1(C_55_Initialization) -> Bus Creator11/1
  Control2/2(C_55_PD_Sort) -> Bus Creator11/2
  Control2/3(C_52_Profibus) -> Bus Creator11/3
  Control2/4(C_55_Start) -> Bus Creator11/4
  Control2/5(C_55_Cart2Del) -> Bus Creator11/5
  Asi/1(A_54_Request) -> Bus Creator10/1
  Asi/2(A_54_No_Cart) -> Bus Creator10/2
  Asi/3(A_54_Cart_Full) -> Bus Creator10/3
  Asi/4(A_54_CRoute_Out) -> Bus Creator10/4
  Asi/5(A_53_SortCartID) -> Bus Creator10/5
  Asi/6(A_54_Cart_Stat) -> Bus Creator10/6
  Asi/7(A_54_Cart_Next) -> Bus Creator10/7
  Asi/8(A_54_Optic) -> Bus Creator10/8
  Asi/9(A_54_Count) -> Bus Creator10/9
  Asi/10(A_54_Pist_Bck) -> Bus Creator10/10
  Asi/11(A_54_Release_FB) -> Bus Creator10/11
  Asi/12(A_54_CRoute_In) -> Bus Creator10/12
  Asi/13(C_55_Start) -> Bus Creator10/13
  Asi/14(C_55_Cart2Del) -> Bus Creator10/14
  Bus Creator10/1 -> Chart/9(AS_i_50)
  Bus Creator11/1 -> Chart/20(Control_50)
  Bus Creator12/1 -> Chart/14(Actuators_50)
  Bus Creator13/1 -> Chart/26(Sensors_50)
  OPC UA Read4/1 -> Bus Selector15/1, Bus Selector14/1, Bus Selector12/1, Bus Selector13/1
  Bus Selector12/1 -> Asi1/1(u1)  "<Value_572>"
  Bus Selector12/2 -> Asi1/2(u2)  "<Value_582>"
  Bus Selector12/3 -> Asi1/3(u3)  "<Value_592>"
  Bus Selector12/4 -> Asi1/4(u4)  "<Value_602>"
  Bus Selector12/5 -> Asi1/5(u5)  "<Value_612>"
  Bus Selector12/6 -> Asi1/6(u6)  "<Value_622>"
  Bus Selector12/7 -> Asi1/7(u7)  "<Value_632>"
  Bus Selector12/8 -> Asi1/8(u8)  "<Value_642>"
  Bus Selector12/9 -> Asi1/9(u9)  "<Value_652>"
  Bus Selector12/10 -> Asi1/10(u10)  "<Value_662>"
  Bus Selector12/11 -> Asi1/11(u11)  "<Value_672>"
  Bus Selector12/12 -> Asi1/12(u12)  "<Value_682>"
  Bus Selector13/1 -> Control3/1(u1)  "<Value_698>"
  Bus Selector13/2 -> Control3/2(u2)  "<Value_708>"
  Bus Selector13/3 -> Control3/3(u3)  "<Value_718>"
  Bus Selector13/4 -> Control3/4(u4)  "<Value_728>"
  Bus Selector13/5 -> Control3/5(u5)  "<Value_738>"
  Bus Selector13/6 -> Control3/6(u6)  "<Value_748>"
  Bus Selector13/7 -> Control3/7(u7)  "<Value_758>"
  Bus Selector14/1 -> Feedback3/1(u1)  "<Value_774>"
  Bus Selector14/2 -> Feedback3/2(u2)  "<Value_784>"
  Bus Selector14/3 -> Feedback3/3(u3)  "<Value_794>"
  Bus Selector14/4 -> Feedback3/4(u4)  "<Value_804>"
  Bus Selector14/5 -> Feedback3/5(u5)  "<Value_814>"
  Bus Selector14/6 -> Feedback3/6(u6)  "<Value_824>"
  Bus Selector14/7 -> Feedback3/7(u7)  "<Value_834>"
  Bus Selector14/8 -> Feedback3/8(u8)  "<Value_844>"
  Bus Selector14/9 -> Feedback3/9(u9)  "<Value_854>"
  Bus Selector14/10 -> Feedback3/10(u10)  "<Value_864>"
  Bus Selector14/11 -> Feedback3/11(u11)  "<Value_874>"
  Bus Selector14/12 -> Feedback3/12(u12)  "<Value_884>"
  Bus Selector15/1 -> Sensors3/1(u1)  "<Value_905>"
  Bus Selector15/2 -> Sensors3/2(u2)  "<Value_918>"
  Bus Selector15/3 -> Sensors3/3(u3)  "<Value_933>"
  Bus Selector15/4 -> Sensors3/4(u4)  "<Value_946>"
  Bus Selector15/5 -> Sensors3/5(u5)  "<Value_959>"
  Bus Selector15/6 -> Sensors3/6(u6)  "<Value_972>"
  Bus Selector15/7 -> Sensors3/7(u7)  "<Value_985>"
  Bus Selector15/8 -> Sensors3/8(u8)  "<Value_998>"
  Bus Selector15/9 -> Sensors3/9(u9)  "<Value_1011>"
  Bus Selector15/10 -> Sensors3/10(u10)  "<Value_1024>"
  Bus Selector15/11 -> Sensors3/11(u11)  "<Value_1037>"
  Bus Selector15/12 -> Sensors3/12(u12)  "<Value_1050>"
  Bus Selector15/13 -> Sensors3/13(u13)  "<Value_1063>"
  Bus Selector15/14 -> Sensors3/14(u14)  "<Value_1076>"
  Bus Selector15/15 -> Sensors3/15(u15)  "<Value_1089>"
  Asi1/1(A_94_Request) -> Bus Creator14/1
  Asi1/2(A_94_No_Cart) -> Bus Creator14/2
  Asi1/3(A_94_Cart_Full) -> Bus Creator14/3
  Asi1/4(A_94_CRoute_Out) -> Bus Creator14/4
  Asi1/5(A_93_ProcCartID) -> Bus Creator14/5
  Asi1/6(A_94_Cart_Stat) -> Bus Creator14/6
  Asi1/7(A_94_Cart_Next) -> Bus Creator14/7
  Asi1/8(A_94_Optic) -> Bus Creator14/8
  Asi1/9(A_94_Count) -> Bus Creator14/9
  Asi1/10(A_94_Pist_Bck) -> Bus Creator14/10
  Asi1/11(A_94_Release_FB) -> Bus Creator14/11
  Asi1/12(A_94_CRoute_In) -> Bus Creator14/12
  Control3/1(C_95_Initialization) -> Bus Creator15/1
  Control3/2(C_95_PD_Proc) -> Bus Creator15/2
  Control3/3(C_95_PD_Cart) -> Bus Creator15/3
  Control3/4(C_92_Profibus) -> Bus Creator15/4
  Control3/5(C_95_Start) -> Bus Creator15/5
  Control3/6(C_95_Cart2Del) -> Bus Creator15/6
  Control3/7(C_95_Del2Cart) -> Bus Creator15/7
  Feedback3/1(F_92_Claw_2_Cart) -> Bus Creator16/1
  Feedback3/2(F_92_Claw_2_Del) -> Bus Creator16/2
  Feedback3/3(F_92_Claw_Down) -> Bus Creator16/3
  Feedback3/4(F_92_Close_Claw) -> Bus Creator16/4
  Feedback3/5(F_93_Led_Start) -> Bus Creator16/5
  Feedback3/6(F_93_Led_Reset) -> Bus Creator16/6
  Feedback3/7(F_93_Led_Extra1) -> Bus Creator16/7
  Feedback3/8(F_93_Led_Extra2) -> Bus Creator16/8
  Feedback3/9(F_93_Panel_O4) -> Bus Creator16/9
  Feedback3/10(F_93_Panel_O5) -> Bus Creator16/10
  Feedback3/11(F_93_Panel_O6) -> Bus Creator16/11
  Feedback3/12(F_93_Panel_O7) -> Bus Creator16/12
  Sensors3/1(O_90_Part_Reserve) -> Bus Creator17/1
  Sensors3/2(O_90_Claw_Del) -> Bus Creator17/2
  Sensors3/3(O_90_Claw_Cart) -> Bus Creator17/3
  Sensors3/4(O_90_Claw_Reserve) -> Bus Creator17/4
  Sensors3/5(O_90_Claw_Low) -> Bus Creator17/5
  Sensors3/6(O_90_Claw_High) -> Bus Creator17/6
  Sensors3/7(O_90_Part_in_Claw) -> Bus Creator17/7
  Sensors3/8(O_91_Start) -> Bus Creator17/8
  Sensors3/9(O_91_Stop) -> Bus Creator17/9
  Sensors3/10(O_91_Key_Pos) -> Bus Creator17/10
  Sensors3/11(O_91_Reset) -> Bus Creator17/11
  Sensors3/12(O_91_Panel_I4) -> Bus Creator17/12
  Sensors3/13(O_91_Panel_I5) -> Bus Creator17/13
  Sensors3/14(O_91_Panel_I6) -> Bus Creator17/14
  Sensors3/15(O_91_Panel_I7) -> Bus Creator17/15
  Bus Creator14/1 -> Chart/10(AS_i_90)
  Bus Creator15/1 -> Chart/22(Control_90)
  Bus Creator16/1 -> Chart/16(Actuators_90)
  Bus Creator17/1 -> Chart/28(Sensors_90)
  Sensors4/1(O_100_PInit_Pos) -> Bus Creator20/1
  Sensors4/2(O_100_PDrill_Pos) -> Bus Creator20/2
  Sensors4/3(O_100_PTest_Pos) -> Bus Creator20/3
  Sensors4/4(O_100_SDrill_High) -> Bus Creator20/4
  Sensors4/5(O_100_SDrill_Low) -> Bus Creator20/5
  Sensors4/6(O_100_RT_Sensor) -> Bus Creator20/6
  Sensors4/7(O_100_PTest_Ok) -> Bus Creator20/7
  Sensors4/8(O_101_Start) -> Bus Creator20/8
  Sensors4/9(O_101_Stop) -> Bus Creator20/9
  Sensors4/10(O_101_Key_Pos) -> Bus Creator20/10
  Sensors4/11(O_101_Reset) -> Bus Creator20/11
  Sensors4/12(O_101_Panel_I4) -> Bus Creator20/12
  Sensors4/13(O_101_Panel_I5) -> Bus Creator20/13
  Sensors4/14(O_101_Panel_I6) -> Bus Creator20/14
  Sensors4/15(O_101_Panel_I7) -> Bus Creator20/15
  Control4/1(C_105_Initialization) -> Bus Creator18/1
  Control4/2(C_105_Part_ready) -> Bus Creator18/2
  Control4/3(C_105_Test_Ok) -> Bus Creator18/3
  Control4/4(C_105_Test_Fail) -> Bus Creator18/4
  Control4/5(C_102_Profibus) -> Bus Creator18/5
  Control4/6(C_103_RQ_Turns) -> Bus Creator18/6
  Control4/7(C_105_Start) -> Bus Creator18/7
  Control4/8(C_105_Test) -> Bus Creator18/8
  Control4/9(C_105_TestDrill) -> Bus Creator18/9
  Control4/10(C_105_Rotation) -> Bus Creator18/10
  Feedback4/1(F_102_Drill_On) -> Bus Creator19/1
  Feedback4/2(F_102_RT_On) -> Bus Creator19/2
  Feedback4/3(F_102_Drill_Down) -> Bus Creator19/3
  Feedback4/4(F_102_Drill_Up) -> Bus Creator19/4
  Feedback4/5(F_102_Drill_Pin) -> Bus Creator19/5
  Feedback4/6(F_102_Test_Pin) -> Bus Creator19/6
  Feedback4/7(F_103_Led_Start) -> Bus Creator19/7
  Feedback4/8(F_103_Led_Reset) -> Bus Creator19/8
  Feedback4/9(F_103_Led_Extra1) -> Bus Creator19/9
  Feedback4/10(F_103_Led_Extra2) -> Bus Creator19/10
  Feedback4/11(F_103_Panel_O4) -> Bus Creator19/11
  Feedback4/12(F_103_Panel_O5) -> Bus Creator19/12
  Feedback4/13(F_103_Panel_O6) -> Bus Creator19/13
  Feedback4/14(F_103_Panel_O7) -> Bus Creator19/14
  Bus Creator18/1 -> Chart/17(Control_100)
  Bus Creator19/1 -> Chart/11(Actuators_100)
  Bus Creator20/1 -> Chart/23(Sensors_100)
  OPC UA Read6/1 -> Bus Selector19/1, Bus Selector17/1, Bus Selector16/1, Bus Selector18/1
  Bus Selector16/1 -> fcn_Asi/1(u1)  "<Value_215>"
  Bus Selector16/2 -> fcn_Asi/2(u2)  "<Value_225>"
  Bus Selector16/3 -> fcn_Asi/3(u3)  "<Value_235>"
  Bus Selector16/4 -> fcn_Asi/4(u4)  "<Value_245>"
  Bus Selector16/5 -> fcn_Asi/5(u5)  "<Value_255>"
  Bus Selector16/6 -> fcn_Asi/6(u6)  "<Value_265>"
  Bus Selector16/7 -> fcn_Asi/7(u7)  "<Value_275>"
  Bus Selector16/8 -> fcn_Asi/8(u8)  "<Value_285>"
  Bus Selector16/9 -> fcn_Asi/9(u9)  "<Value_295>"
  Bus Selector16/10 -> fcn_Asi/10(u10)  "<Value_305>"
  Bus Selector16/11 -> fcn_Asi/11(u11)  "<Value_315>"
  Bus Selector16/12 -> fcn_Asi/12(u12)  "<Value_325>"
  Bus Selector17/1 -> fcn_Control/1(u1)  "<Value_341>"
  Bus Selector17/2 -> fcn_Control/2(u2)  "<Value_354>"
  Bus Selector17/3 -> fcn_Control/3(u3)  "<Value_367>"
  Bus Selector18/1 -> fcn_Feedback/1(u1)  "<Value_383>"
  Bus Selector18/2 -> fcn_Feedback/2(u2)  "<Value_393>"
  Bus Selector18/3 -> fcn_Feedback/3(u3)  "<Value_403>"
  Bus Selector18/4 -> fcn_Feedback/4(u4)  "<Value_413>"
  Bus Selector18/5 -> fcn_Feedback/5(u5)  "<Value_423>"
  Bus Selector18/6 -> fcn_Feedback/6(u6)  "<Value_433>"
  fcn_Asi/1(A_34_Request) -> Bus Creator21/1
  fcn_Asi/2(A_34_No_Cart) -> Bus Creator21/2
  fcn_Asi/3(A_34_Cart_Full) -> Bus Creator21/3
  fcn_Asi/4(A_34_CRoute_Out) -> Bus Creator21/4
  fcn_Asi/5(A_32_RoboCartID) -> Bus Creator21/5
  fcn_Asi/6(A_34_Cart_Stat) -> Bus Creator21/6
  fcn_Asi/7(A_34_Cart_Next) -> Bus Creator21/7
  fcn_Asi/8(A_34_Optic) -> Bus Creator21/8
  fcn_Asi/9(A_34_Count) -> Bus Creator21/9
  fcn_Asi/10(A_34_Pist_Bck) -> Bus Creator21/10
  fcn_Asi/11(A_34_Release_FB) -> Bus Creator21/11
  fcn_Asi/12(A_34_CRoute_In) -> Bus Creator21/12
  fcn_Control/1(C_30_Robot1) -> Bus Creator22/1
  fcn_Control/2(C_30_Robot2) -> Bus Creator22/2
  fcn_Control/3(C_35_Part_Del) -> Bus Creator22/3
  fcn_Feedback/1(F_33_Led_Start) -> Bus Creator23/1
  fcn_Feedback/2(F_33_Led_Reset) -> Bus Creator23/2
  fcn_Feedback/3(F_33_Led_Extra1) -> Bus Creator23/3
  fcn_Feedback/4(F_33_Led_Extra2) -> Bus Creator23/4
  fcn_Feedback/5(F_33_Spring_Cyl) -> Bus Creator23/5
  fcn_Feedback/6(F_33_Cover_Cyl) -> Bus Creator23/6
  fcn_Sensors/1(O_31_Start) -> Bus Creator24/1
  fcn_Sensors/2(O_31_Stop) -> Bus Creator24/2
  fcn_Sensors/3(O_31_Reset) -> Bus Creator24/3
  fcn_Sensors/4(O_31_Part_in_Claw) -> Bus Creator24/4
  fcn_Sensors/5(O_31_Orientation) -> Bus Creator24/5
  fcn_Sensors/6(O_32_Sp_Cyl_Bck) -> Bus Creator24/6
  fcn_Sensors/7(O_32_Sp_Cyl_Fwd) -> Bus Creator24/7
  fcn_Sensors/8(O_32_Co_Cyl_Bck) -> Bus Creator24/8
  fcn_Sensors/9(O_32_Co_Cyl_Fwd) -> Bus Creator24/9
  fcn_Sensors/10(O_32_Sp_PickUp) -> Bus Creator24/10
  fcn_Sensors/11(O_32_Co_PickUp) -> Bus Creator24/11
  fcn_Sensors/12(O_32_CoMag_Empty) -> Bus Creator24/12
  Bus Creator21/1 -> Chart/8(AS_i_30)
  Bus Creator22/1 -> Chart/19(Control_30)
  Bus Creator23/1 -> Chart/13(Actuators_30)
  Bus Creator24/1 -> Chart/25(Sensors_30)
  OPC UA Read7/1 -> Bus Selector22/1, Bus Selector20/1, Bus Selector21/1
  Bus Selector20/1 -> Control5/1(u1)  "<Value_566>"
  Bus Selector20/2 -> Control5/2(u2)  "<Value_576>"
  Bus Selector20/3 -> Control5/3(u3)  "<Value_586>"
  Bus Selector20/4 -> Control5/4(u4)  "<Value_596>"
  Bus Selector20/5 -> Control5/5(u5)  "<Value_606>"
  Bus Selector20/6 -> Control5/6(u6)  "<Value_616>"
  Bus Selector20/7 -> Control5/7(u7)  "<Value_626>"
  Bus Selector20/8 -> Control5/8(u8)  "<Value_636>"
  Bus Selector20/9 -> Control5/9(u9)  "<Value_646>"
  Bus Selector20/10 -> Control5/10(u10)  "<Value_656>"
  Bus Selector20/11 -> Control5/11(u11)  "<Value_666>"
  Bus Selector21/1 -> Feedback5/1(u1)  "<Value_682>"
  Bus Selector21/2 -> Feedback5/2(u2)  "<Value_692>"
  Bus Selector21/3 -> Feedback5/3(u3)  "<Value_702>"
  Bus Selector21/4 -> Feedback5/4(u4)  "<Value_712>"
  Bus Selector21/5 -> Feedback5/5(u5)  "<Value_722>"
  Bus Selector21/6 -> Feedback5/6(u6)  "<Value_732>"
  Bus Selector21/7 -> Feedback5/7(u7)  "<Value_742>"
  Bus Selector21/8 -> Feedback5/8(u8)  "<Value_752>"
  Bus Selector21/9 -> Feedback5/9(u9)  "<Value_762>"
  Bus Selector21/10 -> Feedback5/10(u10)  "<Value_772>"
  Bus Selector21/11 -> Feedback5/11(u11)  "<Value_782>"
  Bus Selector21/12 -> Feedback5/12(u12)  "<Value_792>"
  Bus Selector22/1 -> Sensors5/1(u1)  "<Value_811>"
  Bus Selector22/2 -> Sensors5/2(u2)  "<Value_824>"
  Bus Selector22/3 -> Sensors5/3(u3)  "<Value_839>"
  Bus Selector22/4 -> Sensors5/4(u4)  "<Value_852>"
  Bus Selector22/5 -> Sensors5/5(u5)  "<Value_865>"
  Bus Selector22/6 -> Sensors5/6(u6)  "<Value_878>"
  Bus Selector22/7 -> Sensors5/7(u7)  "<Value_891>"
  Bus Selector22/8 -> Sensors5/8(u8)  "<Value_904>"
  Bus Selector22/9 -> Sensors5/9(u9)  "<Value_917>"
  Bus Selector22/10 -> Sensors5/10(u10)  "<Value_930>"
  Bus Selector22/11 -> Sensors5/11(u11)  "<Value_943>"
  Bus Selector22/12 -> Sensors5/12(u12)  "<Value_956>"
  Bus Selector22/13 -> Sensors5/13(u13)  "<Value_969>"
  Bus Selector22/14 -> Sensors5/14(u14)  "<Value_982>"
  Bus Selector22/15 -> Sensors5/15(u15)  "<Value_995>"
  Bus Selector22/16 -> Sensors5/16(u16)  "<Value_1008>"
  Control5/1(C_65_Initialization) -> Bus Creator25/1
  Control5/2(C_65_ID_1) -> Bus Creator25/2
  Control5/3(C_65_ID_2) -> Bus Creator25/3
  Control5/4(C_65_Part_Sorted) -> Bus Creator25/4
  Control5/5(C_62_Profibus) -> Bus Creator25/5
  Control5/6(C_65_RBS_Output) -> Bus Creator25/6
  Control5/7(C_65_RSB_Output) -> Bus Creator25/7
  Control5/8(C_65_BRS_Output) -> Bus Creator25/8
  Control5/9(C_65_BSR_Output) -> Bus Creator25/9
  Control5/10(C_65_SRB_Output) -> Bus Creator25/10
  Control5/11(C_65_SBR_Output) -> Bus Creator25/11
  Feedback5/1(F_62_Conveyor) -> Bus Creator26/1
  Feedback5/2(F_62_P1) -> Bus Creator26/2
  Feedback5/3(F_62_P2) -> Bus Creator26/3
  Feedback5/4(F_62_Identify) -> Bus Creator26/4
  Feedback5/5(F_63_Led_Start) -> Bus Creator26/5
  Feedback5/6(F_63_Led_Reset) -> Bus Creator26/6
  Feedback5/7(F_63_Led_Extra1) -> Bus Creator26/7
  Feedback5/8(F_63_Led_Extra2) -> Bus Creator26/8
  Feedback5/9(F_63_Panel_O4) -> Bus Creator26/9
  Feedback5/10(F_63_Panel_O5) -> Bus Creator26/10
  Feedback5/11(F_63_Panel_O6) -> Bus Creator26/11
  Feedback5/12(F_63_Panel_O7) -> Bus Creator26/12
  Sensors5/1(O_60_SPart) -> Bus Creator27/1
  Sensors5/2(O_60_Slnd) -> Bus Creator27/2
  Sensors5/3(O_60_SPhoto) -> Bus Creator27/3
  Sensors5/4(O_60_Part_Pass) -> Bus Creator27/4
  Sensors5/5(O_60_SL1_Bck) -> Bus Creator27/5
  Sensors5/6(O_60_SL1_Fwd) -> Bus Creator27/6
  Sensors5/7(O_60_SL2_Bck) -> Bus Creator27/7
  Sensors5/8(O_60_SL2_Fwd) -> Bus Creator27/8
  Sensors5/9(O_61_Start) -> Bus Creator27/9
  Sensors5/10(O_61_Stop) -> Bus Creator27/10
  Sensors5/11(O_61_Key_Pos) -> Bus Creator27/11
  Sensors5/12(O_61_Reset) -> Bus Creator27/12
  Sensors5/13(O_61_Panel_I4) -> Bus Creator27/13
  Sensors5/14(O_61_Panel_I5) -> Bus Creator27/14
  Sensors5/15(O_61_Panel_I6) -> Bus Creator27/15
  Sensors5/16(O_61_Panel_I7) -> Bus Creator27/16
  Bus Creator25/1 -> Chart/21(Control_60)
  Bus Creator26/1 -> Chart/15(Actuators_60)
  Bus Creator27/1 -> Chart/27(Sensors_60)
